simulink model "capitol6prob4"  (R2013a)
settings: Solver=ode45  StartTime=0.0  StopTime=3600  RelTol=1e-3
undefined symbols (not defined in the file): des, gcbh
settings Model: Creator=user  LastModifiedBy=user

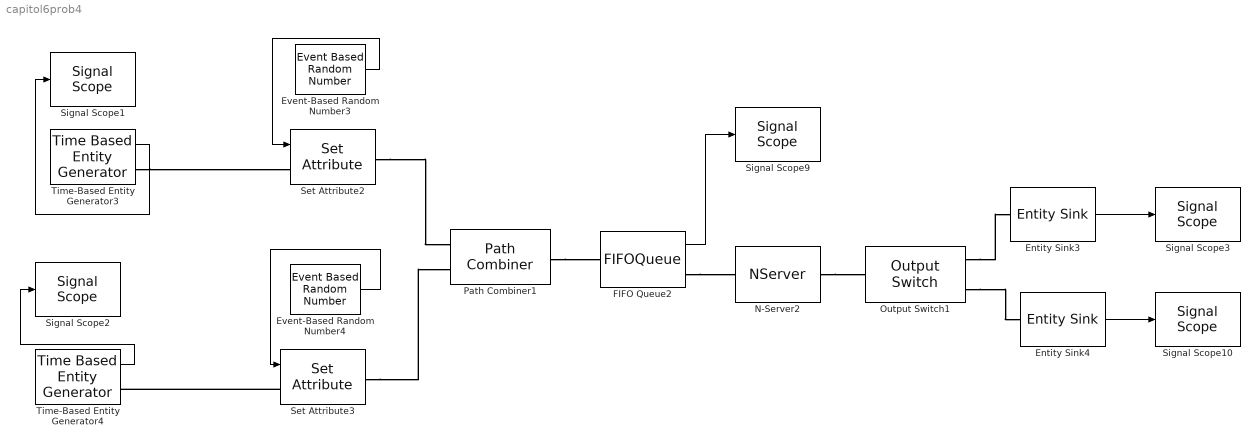
== system capitol6prob4 ==
  Entity Sink3 : EntitySink  StatNumberArrived=on
  Entity Sink4 : EntitySink  StatNumberArrived=on
  Event-Based Random Number3 : EventBasedRandomNumber  Distribution=Uniform  minUnif=21  maxUnif=39  Seed=1234567
  Event-Based Random Number4 : EventBasedRandomNumber  Distribution=Uniform  minUnif=9  maxUnif=15  Seed=12345678
  FIFO Queue2 : FIFOQueue  StatAverageQueueLength=on
      settings: OutputPortMap=o3
  N-Server2 : NServer  NumberOfServers=2  ServiceTimeFrom=Attribute
  Output Switch1 : OutputSwitch  NumberOutputPorts=2  SwitchingCriterion=From attribute  AttributeName=Muncitor
  Path Combiner1 : PathCombiner  NumberInputPorts=2
  Set Attribute2 : SetAttribute  AttributeName=ServiceTime|Muncitor  AttributeFrom=Signal port|Dialog  AttributeValue=1|1  AttributeTreatAsVector=1|1  EvaluatedAttributeValue={ [];1}
  Set Attribute3 : SetAttribute  AttributeName=ServiceTime|Muncitor  AttributeFrom=Signal port|Dialog  AttributeValue=1|2  AttributeTreatAsVector=1|1  EvaluatedAttributeValue={ [];2}
  Signal Scope{1..3,9..10} (5 alike) : SignalScope  LoadFcn=des.scope.CallbackSupport('seLoadFcn',gcbh)  StartFcn=des.scope.CallbackSupport('seStartFcn',gcbh)  StopFcn=des.scope.CallbackSupport('seStopFcn',gcbh)
      settings: CopyFcn=des.scope.CallbackSupport('seCopyFcn',gcbh)  DeleteFcn=des.scope.CallbackSupport('seDeleteFcn',gcbh)  PreSaveFcn=des.scope.CallbackSupport('sePreSaveFcn',gcbh)  NameChangeFcn=des.scope.CallbackSupport('seNameChangeFcn',gcbh)  OpenFcn=des.scope.CallbackSupport('seOpenFcn',gcbh)
  Time-Based Entity Generator3 : TimeBasedEntityGenerator  Distribution=Uniform  Minimum=39  Maximum=45  Mean=0.2  StatNumberDeparted=on
  Time-Based Entity Generator4 : TimeBasedEntityGenerator  Distribution=Uniform  InitialSeed=123456  Minimum=40  Maximum=60  Mean=0.2  StatNumberDeparted=on
  wires:
  FIFO Queue2/1 -> Signal Scope9/1
  Event-Based Random Number4/1 -> Set Attribute3/1
  Event-Based Random Number3/1 -> Set Attribute2/1
  Time-Based Entity Generator3/1 -> Signal Scope1/1
  Time-Based Entity Generator4/1 -> Signal Scope2/1
  Entity Sink3/1 -> Signal Scope3/1
  Entity Sink4/1 -> Signal Scope10/1
  connections:
  Output Switch1/RConn1 -- Entity Sink3/LConn1
  Set Attribute2/RConn1 -- Path Combiner1/LConn1
  Output Switch1/RConn2 -- Entity Sink4/LConn1
  Time-Based Entity Generator3/RConn1 -- Set Attribute2/LConn1
  Path Combiner1/RConn1 -- FIFO Queue2/LConn1
  N-Server2/RConn1 -- Output Switch1/LConn1
  FIFO Queue2/RConn1 -- N-Server2/LConn1
  Set Attribute3/RConn1 -- Path Combiner1/LConn2
  Set Attribute3/LConn1 -- Time-Based Entity Generator4/RConn1
